simulink model "sedemo_mod_markov_poisson"  (Simulink 7.5)
settings: Solver=VariableStepDiscrete  StartTime=0.0  StopTime=200  MaxStep=inf  RelTol=1e-3
libraries: simeventssink1 x10, simeventsgenerators1 x6, simulink x3, simeventsgates1 x3, simeventstranslate1 x3, simeventsinfo x1, simeventsrouting1 x1
settings Model: Creator=The MathWorks Inc.  ExtModeAutoUpdateStatusClock=off
settings DataIOCC: SaveOutput=off  SignalLogging=off  SaveTime=off
settings OptimizationCC: InitFltsAndDblsToZero=on
settings DebuggingCC: AlgebraicLoopMsg=error  SignalResolutionControl=TryResolveAllWithWarning  SolverPrmCheckMsg=none  MultiTaskDSMMsg=warning  StrictBusMsg=Warning
settings SimEventsCC: propDiagAttribOutput=1  propDiagFcnCallOutput=1  propDiagStatOutput=0

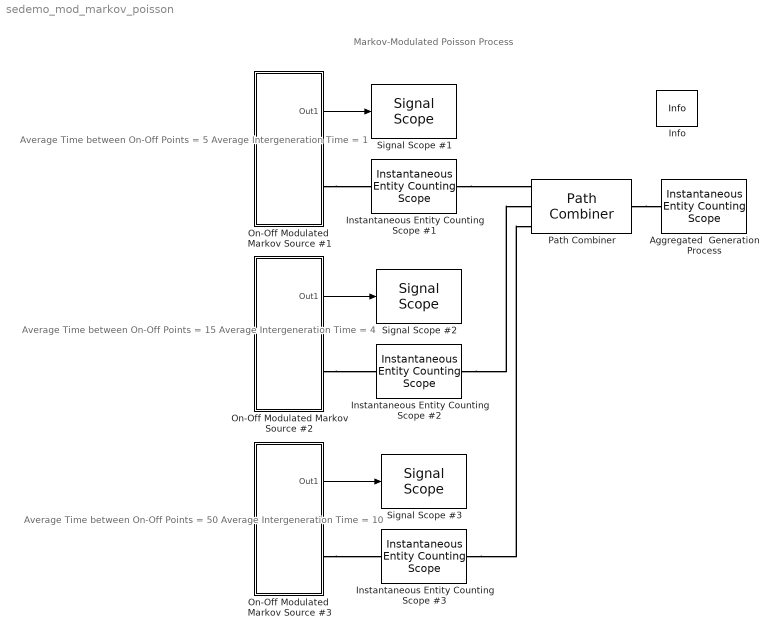
== system sedemo_mod_markov_poisson ==
  note: Markov-Modulated Poisson Process
  note: Average Time
      | between On-Off
      | Points = 5
      |
      | Average
      | Intergeneration
      | Time = 1
  note: Average Time
      | between On-Off
      | Points = 15
      |
      | Average
      | Intergeneration
      | Time = 4
  note: Average Time
      | between On-Off
      | Points = 50
      |
      | Average
      | Intergeneration
      | Time = 10
  Aggregated  Generation Process : simeventssink1/Instantaneous Entity Counting Scope  Priority=1  SystemSampleTime=-1  PlotType=Instantaneous entity counting  InputType=Attribute  NumInputs=1  AttributeNameY=Count  XInputOptionSignal=Event time  XInputOptionEntity=Event time  AttributeNameX=Count  EnableEntityOutport=off  XMin=-1.99963192867081  XMax=202  XLimitExceededOption=Stretch axis limits  YLimitExceededOption=Stretch axis limits  AxisGrid=on  AxisLegend=off  LineDisables=""  LineColors=b  LineStyles=-  LineMarkers=.  OpenScopeAtSimStart=on  Title=Aggregated Entity Generation  YLabel=Entity Generation Points  XLabel=Time  FigurePosition=[697 423 303 214]  AxisZoom=off  DataStoreOption=Limited  DataPointsLimit=10000  StatNumberArrived=Off  ShowCountPlotted=off  ShowToolbar=on
      settings: YMin=-0.02  YMax=1.1
  Info : simeventsinfo/Info  SystemSampleTime=-1
  Instantaneous Entity Counting Scope #1 : simeventssink1/Instantaneous Entity Counting Scope  Priority=1  SystemSampleTime=-1  PlotType=Instantaneous entity counting  InputType=Attribute  NumInputs=1  AttributeNameY=Count  XInputOptionSignal=Event time  XInputOptionEntity=Event time  AttributeNameX=Count  EnableEntityOutport=on  XMin=-1.99963192867081  XMax=202  XLimitExceededOption=Stretch axis limits  YLimitExceededOption=Stretch axis limits  AxisGrid=on  AxisLegend=off  LineDisables=""  LineColors=b  LineStyles=-  LineMarkers=.  OpenScopeAtSimStart=on  Title=Modulated Entity Generation #1  YLabel=Generation Points  XLabel=Time  FigurePosition=[320 505 372 139]  AxisZoom=off  DataStoreOption=Limited  DataPointsLimit=10000  StatNumberArrived=Off  ShowCountPlotted=off  ShowToolbar=off
      settings: YMin=-0.02  YMax=1.1
  Instantaneous Entity Counting Scope #2 : simeventssink1/Instantaneous Entity Counting Scope  Priority=1  SystemSampleTime=-1  PlotType=Instantaneous entity counting  InputType=Attribute  NumInputs=1  AttributeNameY=Count  XInputOptionSignal=Event time  XInputOptionEntity=Event time  AttributeNameX=Count  EnableEntityOutport=on  XMin=-1.9001134042793  XMax=202  XLimitExceededOption=Stretch axis limits  YLimitExceededOption=Stretch axis limits  AxisGrid=on  AxisLegend=off  LineDisables=""  LineColors=b  LineStyles=-  LineMarkers=.  OpenScopeAtSimStart=on  Title=Modulated Entity Generation #2  YLabel=Generation Points  XLabel=Time  FigurePosition=[320 686 371 140]  AxisZoom=off  DataStoreOption=Limited  DataPointsLimit=10000  StatNumberArrived=Off  ShowCountPlotted=off  ShowToolbar=off
      settings: YMin=-0.02  YMax=1.1
  Instantaneous Entity Counting Scope #3 : simeventssink1/Instantaneous Entity Counting Scope  Priority=1  SystemSampleTime=-1  PlotType=Instantaneous entity counting  InputType=Attribute  NumInputs=1  AttributeNameY=Count  XInputOptionSignal=Event time  XInputOptionEntity=Event time  AttributeNameX=Count  EnableEntityOutport=on  XMin=-1.75311680759808  XMax=202  XLimitExceededOption=Stretch axis limits  YLimitExceededOption=Stretch axis limits  AxisGrid=on  AxisLegend=off  LineDisables=""  LineColors=b  LineStyles=-  LineMarkers=.  OpenScopeAtSimStart=on  Title=Modulated Entity Generation #3  YLabel=Generation Points  XLabel=Time  FigurePosition=[321 330 370 138]  AxisZoom=off  DataStoreOption=Limited  DataPointsLimit=10000  StatNumberArrived=Off  ShowCountPlotted=off  ShowToolbar=off
      settings: YMin=-0.02  YMax=1.1
  On-Off Modulated Markov Source #2 : Subsystem
  On-Off Modulated  Markov Source #1 : Subsystem
  On-Off Modulated  Markov Source #3 : Subsystem
  Path Combiner : simeventsrouting1/Path Combiner  Priority=1  SystemSampleTime=-1  NumberInputPorts=3  InputPortPrecedence=IN1 port  InitialSeed=45675  SpecifyEventPriority=off  PriorityPathCombinerPortPrecedenceSelection=4100  StatNumberDeparted=Off  StatLastArrivalPort=Off  EvaluatedNumPorts=3
  Signal Scope #1 : simeventssink1/Signal Scope  Priority=1  SystemSampleTime=-1  PlotType=Stair  InputType=Signal  NumInputs=1  AttributeNameY=Count  XInputOptionSignal=Event time  XInputOptionEntity=Event time  AttributeNameX=Count  EnableEntityOutport=on  XMin=-1.95  XMax=202  XLimitExceededOption=Stretch axis limits  YLimitExceededOption=Stretch axis limits  AxisGrid=on  AxisLegend=off  LineDisables=""  LineColors=b  LineStyles=-  LineMarkers=None  OpenScopeAtSimStart=on  Title=On-Off Process #1  YLabel=Enable  XLabel=Time  FigurePosition=[11 685 301 142]  AxisZoom=off  DataStoreOption=Limited  DataPointsLimit=10000  StatNumberArrived=Off  ShowCountPlotted=off  ShowToolbar=off
      settings: YMin=-0.02  YMax=1.1
  Signal Scope #2 : simeventssink1/Signal Scope  Priority=1  SystemSampleTime=-1  PlotType=Stair  InputType=Signal  NumInputs=1  AttributeNameY=Count  XInputOptionSignal=Event time  XInputOptionEntity=Event time  AttributeNameX=Count  EnableEntityOutport=on  XMin=-1.99544522692409  XMax=202  XLimitExceededOption=Stretch axis limits  YLimitExceededOption=Stretch axis limits  AxisGrid=on  AxisLegend=off  LineDisables=""  LineColors=b  LineStyles=-  LineMarkers=None  OpenScopeAtSimStart=on  Title=On-Off Process #2  YLabel=Enable  XLabel=Time  FigurePosition=[10 506 302 139]  AxisZoom=off  DataStoreOption=Limited  DataPointsLimit=10000  StatNumberArrived=Off  ShowCountPlotted=off  ShowToolbar=off
      settings: YMin=-0.01  YMax=1.1
  Signal Scope #3 : simeventssink1/Signal Scope  Priority=1  SystemSampleTime=-1  PlotType=Stair  InputType=Signal  NumInputs=1  AttributeNameY=Count  XInputOptionSignal=Event time  XInputOptionEntity=Event time  AttributeNameX=Count  EnableEntityOutport=on  XMin=0  XMax=202  XLimitExceededOption=Stretch axis limits  YLimitExceededOption=Stretch axis limits  AxisGrid=on  AxisLegend=off  LineDisables=""  LineColors=b  LineStyles=-  LineMarkers=None  OpenScopeAtSimStart=on  Title=On-Off Process #3  YLabel=Enable  XLabel=Time  FigurePosition=[8 330 303 139]  AxisZoom=off  DataStoreOption=Limited  DataPointsLimit=10000  StatNumberArrived=Off  ShowCountPlotted=off  ShowToolbar=off
      settings: YMin=-0.01  YMax=1.1
  wires:
  On-Off Modulated  Markov Source #1/1(Out1) -> Signal Scope #1/1
  On-Off Modulated Markov Source #2/1(Out1) -> Signal Scope #2/1
  On-Off Modulated  Markov Source #3/1(Out1) -> Signal Scope #3/1
  connections:
  On-Off Modulated  Markov Source #1/RConn1 -- Instantaneous Entity Counting Scope #1/LConn1
  On-Off Modulated Markov Source #2/RConn1 -- Instantaneous Entity Counting Scope #2/LConn1
  On-Off Modulated  Markov Source #3/RConn1 -- Instantaneous Entity Counting Scope #3/LConn1
  Instantaneous Entity Counting Scope #1/RConn1 -- Path Combiner/LConn1
  Instantaneous Entity Counting Scope #2/RConn1 -- Path Combiner/LConn2
  Instantaneous Entity Counting Scope #3/RConn1 -- Path Combiner/LConn3
  Path Combiner/RConn1 -- Aggregated  Generation Process/LConn1

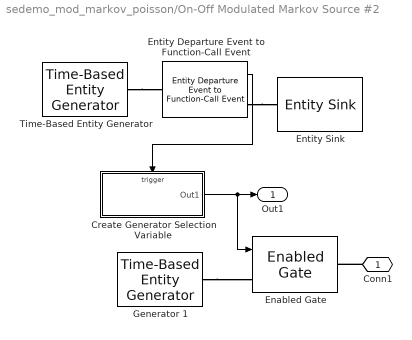
== system sedemo_mod_markov_poisson/On-Off Modulated Markov Source #2 ==
  Create Generator Selection Variable : Subsystem  TreatAsAtomicUnit=on
      settings: PropExecContextOutsideSubsystem=on
  Enabled Gate : simeventsgates1/Enabled Gate  Priority=1  SystemSampleTime=-1  SpecifyEventPriority=off  PriorityGateEnableOpenClose=2000  StatNumberDeparted=Off
  Entity Departure Event to Function-Call Event : simeventstranslate1/Entity Departure Event to Function-Call Event  Priority=1  SystemSampleTime=-1  TimingFunctionCallF1=After entity departure  EnableE1Port=off  EnableF2Port=off  TimingFunctionCallF2=Before entity departure  EnableE2Port=off  StatNumberDeparted=Off  StatNumberF1Calls=Off  StatNumberF2Calls=Off  IsInsideAFB=off
  Entity Sink : simeventssink1/Entity Sink  Priority=1  SystemSampleTime=-1  AvailableForArrivals=on  StatNumberArrived=Off
  Generator 1 : simeventsgenerators1/Entity Generators/Time-Based Entity Generator  Priority=1  DialogController=des_ddg_create  DialogControllerArgs=DataTag8  SystemSampleTime=-1  GenerateEntitiesUpon=Intergeneration time from dialog  Distribution=Exponential  Minimum=0  Maximum=.2  Mean=4  InitialSeed=54323  Period=.1  PriorityEntityGeneration=300  GenerateEntityAtSimulationStart=on  ResponseWhenBlocked=Pause generation  ResponseWhenUnblocked=Delayed restart  EntityType=Standard  StatNumberDeparted=Off  StatPendingEntity=Off  StatAverageIntergenerationTime=Off
  Time-Based Entity Generator : simeventsgenerators1/Entity Generators/Time-Based Entity Generator  Priority=1  DialogController=des_ddg_create  DialogControllerArgs=DataTag10  SystemSampleTime=-1  GenerateEntitiesUpon=Intergeneration time from dialog  Distribution=Exponential  Minimum=0  Maximum=2  Mean=15  InitialSeed=22345  Period=15  PriorityEntityGeneration=350  GenerateEntityAtSimulationStart=on  ResponseWhenBlocked=Pause generation  ResponseWhenUnblocked=Immediate restart  EntityType=Standard  StatNumberDeparted=Off  StatPendingEntity=Off  StatAverageIntergenerationTime=Off
  Conn1 : PMIOPort  Port=1  Side=Right
  Out1 : Outport  OutDataType=sfix(16)  OutScaling=2^0
  wires:
  Entity Departure Event to Function-Call Event/1 -> Create Generator Selection Variable/Trigger
  Create Generator Selection Variable/1(Out1) -> Enabled Gate/1, Out1/1
  connections:
  Generator 1/RConn1 -- Enabled Gate/LConn1
  Time-Based Entity Generator/RConn1 -- Entity Departure Event to Function-Call Event/LConn1
  Entity Departure Event to Function-Call Event/RConn1 -- Entity Sink/LConn1
  Conn1/RConn1 -- Enabled Gate/RConn1

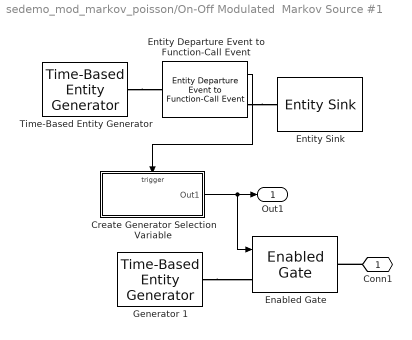
== system sedemo_mod_markov_poisson/On-Off Modulated  Markov Source #1 ==
  Create Generator Selection Variable : Subsystem  TreatAsAtomicUnit=on
      settings: PropExecContextOutsideSubsystem=on
  Enabled Gate : simeventsgates1/Enabled Gate  Priority=1  SystemSampleTime=-1  SpecifyEventPriority=off  PriorityGateEnableOpenClose=2000  StatNumberDeparted=Off
  Entity Departure Event to Function-Call Event : simeventstranslate1/Entity Departure Event to Function-Call Event  Priority=1  SystemSampleTime=-1  TimingFunctionCallF1=After entity departure  EnableE1Port=off  EnableF2Port=off  TimingFunctionCallF2=Before entity departure  EnableE2Port=off  StatNumberDeparted=Off  StatNumberF1Calls=Off  StatNumberF2Calls=Off  IsInsideAFB=off
  Entity Sink : simeventssink1/Entity Sink  Priority=1  SystemSampleTime=-1  AvailableForArrivals=on  StatNumberArrived=Off
  Generator 1 : simeventsgenerators1/Entity Generators/Time-Based Entity Generator  Priority=1  DialogController=des_ddg_create  DialogControllerArgs=DataTag15  SystemSampleTime=-1  GenerateEntitiesUpon=Intergeneration time from dialog  Distribution=Exponential  Minimum=0  Maximum=.2  Mean=1  InitialSeed=54321  Period=.1  PriorityEntityGeneration=300  GenerateEntityAtSimulationStart=on  ResponseWhenBlocked=Pause generation  ResponseWhenUnblocked=Delayed restart  EntityType=Standard  StatNumberDeparted=Off  StatPendingEntity=Off  StatAverageIntergenerationTime=Off
  Time-Based Entity Generator : simeventsgenerators1/Entity Generators/Time-Based Entity Generator  Priority=1  DialogController=des_ddg_create  DialogControllerArgs=DataTag17  SystemSampleTime=-1  GenerateEntitiesUpon=Intergeneration time from dialog  Distribution=Exponential  Minimum=0  Maximum=2  Mean=5  InitialSeed=12345  Period=15  PriorityEntityGeneration=350  GenerateEntityAtSimulationStart=on  ResponseWhenBlocked=Pause generation  ResponseWhenUnblocked=Immediate restart  EntityType=Standard  StatNumberDeparted=Off  StatPendingEntity=Off  StatAverageIntergenerationTime=Off
  Conn1 : PMIOPort  Port=1  Side=Right
  Out1 : Outport  OutDataType=sfix(16)  OutScaling=2^0
  wires:
  Entity Departure Event to Function-Call Event/1 -> Create Generator Selection Variable/Trigger
  Create Generator Selection Variable/1(Out1) -> Enabled Gate/1, Out1/1
  connections:
  Generator 1/RConn1 -- Enabled Gate/LConn1
  Time-Based Entity Generator/RConn1 -- Entity Departure Event to Function-Call Event/LConn1
  Entity Departure Event to Function-Call Event/RConn1 -- Entity Sink/LConn1
  Conn1/RConn1 -- Enabled Gate/RConn1

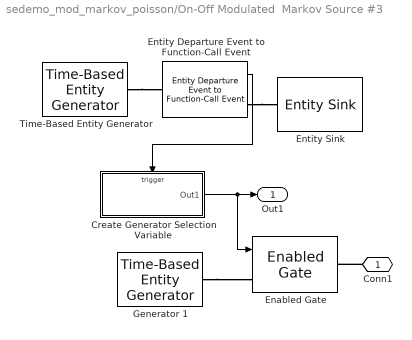
== system sedemo_mod_markov_poisson/On-Off Modulated  Markov Source #3 ==
  Create Generator Selection Variable : Subsystem  TreatAsAtomicUnit=on
      settings: PropExecContextOutsideSubsystem=on
  Enabled Gate : simeventsgates1/Enabled Gate  Priority=1  SystemSampleTime=-1  SpecifyEventPriority=off  PriorityGateEnableOpenClose=2000  StatNumberDeparted=Off
  Entity Departure Event to Function-Call Event : simeventstranslate1/Entity Departure Event to Function-Call Event  Priority=1  SystemSampleTime=-1  TimingFunctionCallF1=After entity departure  EnableE1Port=off  EnableF2Port=off  TimingFunctionCallF2=Before entity departure  EnableE2Port=off  StatNumberDeparted=Off  StatNumberF1Calls=Off  StatNumberF2Calls=Off  IsInsideAFB=off
  Entity Sink : simeventssink1/Entity Sink  Priority=1  SystemSampleTime=-1  AvailableForArrivals=on  StatNumberArrived=Off
  Generator 1 : simeventsgenerators1/Entity Generators/Time-Based Entity Generator  Priority=1  DialogController=des_ddg_create  DialogControllerArgs=DataTag22  SystemSampleTime=-1  GenerateEntitiesUpon=Intergeneration time from dialog  Distribution=Exponential  Minimum=0  Maximum=.2  Mean=10  InitialSeed=54325  Period=.1  PriorityEntityGeneration=300  GenerateEntityAtSimulationStart=on  ResponseWhenBlocked=Pause generation  ResponseWhenUnblocked=Delayed restart  EntityType=Standard  StatNumberDeparted=Off  StatPendingEntity=Off  StatAverageIntergenerationTime=Off
  Time-Based Entity Generator : simeventsgenerators1/Entity Generators/Time-Based Entity Generator  Priority=1  DialogController=des_ddg_create  DialogControllerArgs=DataTag24  SystemSampleTime=-1  GenerateEntitiesUpon=Intergeneration time from dialog  Distribution=Exponential  Minimum=0  Maximum=2  Mean=50  InitialSeed=32345  Period=15  PriorityEntityGeneration=350  GenerateEntityAtSimulationStart=on  ResponseWhenBlocked=Pause generation  ResponseWhenUnblocked=Immediate restart  EntityType=Standard  StatNumberDeparted=Off  StatPendingEntity=Off  StatAverageIntergenerationTime=Off
  Conn1 : PMIOPort  Port=1  Side=Right
  Out1 : Outport  OutDataType=sfix(16)  OutScaling=2^0
  wires:
  Entity Departure Event to Function-Call Event/1 -> Create Generator Selection Variable/Trigger
  Create Generator Selection Variable/1(Out1) -> Enabled Gate/1, Out1/1
  connections:
  Generator 1/RConn1 -- Enabled Gate/LConn1
  Time-Based Entity Generator/RConn1 -- Entity Departure Event to Function-Call Event/LConn1
  Entity Departure Event to Function-Call Event/RConn1 -- Entity Sink/LConn1
  Conn1/RConn1 -- Enabled Gate/RConn1

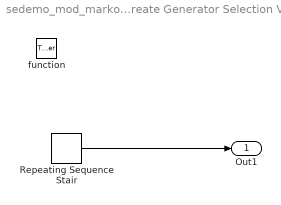
== system sedemo_mod_markov_poisson/On-Off Modulated Markov Source #2/Create Generator Selection Variable ==
  function : TriggerPort  TriggerType=function-call
  Repeating Sequence Stair : simulink/Sources/Repeating Sequence Stair  SystemSampleTime=-1  OutValues=[0 1].'  tsamp=-1  OutputDataTypeScalingMode=Specify via dialog  OutDataType=float('double')  ConRadixGroup=Best Precision: Vector-wise  OutScaling=2^-12
  Out1 : Outport  OutDataType=sfix(16)  OutScaling=2^0
  wires:
  Repeating Sequence Stair/1 -> Out1/1

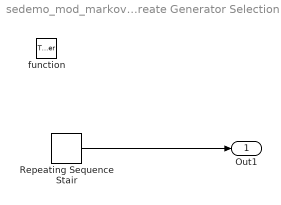
== system sedemo_mod_markov_poisson/On-Off Modulated  Markov Source #1/Create Generator Selection Variable ==
  function : TriggerPort  TriggerType=function-call
  Repeating Sequence Stair : simulink/Sources/Repeating Sequence Stair  SystemSampleTime=-1  OutValues=[0 1].'  tsamp=-1  OutputDataTypeScalingMode=Specify via dialog  OutDataType=float('double')  ConRadixGroup=Best Precision: Vector-wise  OutScaling=2^-12
  Out1 : Outport  OutDataType=sfix(16)  OutScaling=2^0
  wires:
  Repeating Sequence Stair/1 -> Out1/1

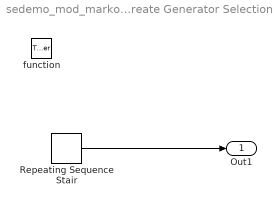
== system sedemo_mod_markov_poisson/On-Off Modulated  Markov Source #3/Create Generator Selection Variable ==
  function : TriggerPort  TriggerType=function-call
  Repeating Sequence Stair : simulink/Sources/Repeating Sequence Stair  SystemSampleTime=-1  OutValues=[0 1].'  tsamp=-1  OutputDataTypeScalingMode=Specify via dialog  OutDataType=float('double')  ConRadixGroup=Best Precision: Vector-wise  OutScaling=2^-12
  Out1 : Outport  OutDataType=sfix(16)  OutScaling=2^0
  wires:
  Repeating Sequence Stair/1 -> Out1/1
